simulink model "motorSIM"  (R2015a)
settings: Solver=ode45  StartTime=0.0  StopTime=10.0  RelTol=1e-3
values from neighbouring files (symbols this model uses):
  b = 0.1    [motor.m]    (also in spring_damper.m = 2)
  j = 0.01    [motor.m]
  k = 0.01    [motor.m]    (also in spring_damper.m = 1)
  L = 0.5    [motor.m]
  R = 1    [motor.m]
  vi = 6    [motor.m]
settings Model: Creator=ahmed alaa  LastModifiedBy=ahmed alaa

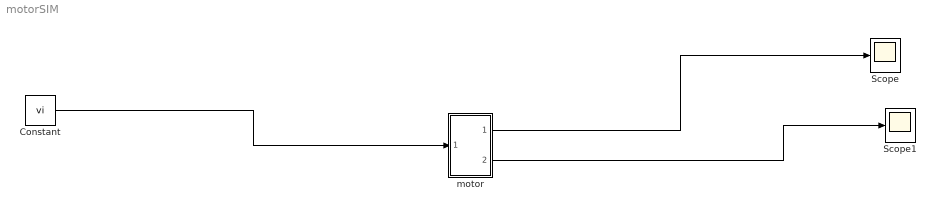
== system motorSIM ==
  Constant : Constant  Value=vi
  Scope : Scope
  Scope1 : Scope
  motor : Subsystem
  wires:
  Constant/1 -> motor/1(volt)
  motor/1(Out1) -> Scope/1
  motor/2(Out2) -> Scope1/1

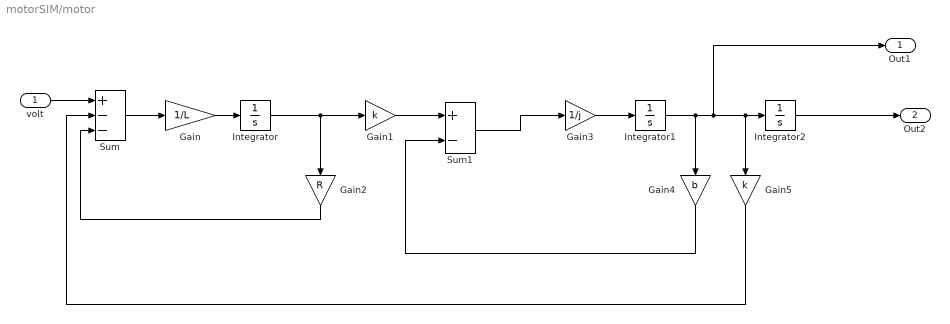
== system motorSIM/motor ==
  volt : Inport
  Gain : Gain  Gain=1/L
  Gain1 : Gain  Gain=k
  Gain2 : Gain  Gain=R
  Gain3 : Gain  Gain=1/j
  Gain4 : Gain  Gain=b
  Gain5 : Gain  Gain=k
  Integrator : Integrator
  Integrator1 : Integrator
  Integrator2 : Integrator
  Sum : Sum  Inputs=+--
  Sum1 : Sum  Inputs=+-
  Out1 : Outport
  Out2 : Outport  Port=2
  wires:
  Gain/1 -> Integrator/1
  Gain3/1 -> Integrator1/1
  Integrator1/1 -> Out1/1, Integrator2/1, Gain5/1, Gain4/1
  Gain2/1 -> Sum/3
  Sum1/1 -> Gain3/1
  volt/1 -> Sum/1
  Gain5/1 -> Sum/2
  Sum/1 -> Gain/1
  Gain4/1 -> Sum1/2
  Integrator2/1 -> Out2/1
  Integrator/1 -> Gain1/1, Gain2/1
  Gain1/1 -> Sum1/1
